simulink model "mdl4"  (Simulink 8.3)
settings: Solver=FixedStepDiscrete  SolverMode=SingleTasking  StartTime=TIME(1)  StopTime=TIME(end)  FixedStep=SIMSTEP  RelTol=1e-3
values from neighbouring files (symbols this model uses):
  Parameter113 = 123    [scr_simdata_all.mat]
  Parameter131 = 3    [scr_simdata_all.mat]
  Parameter132 = 100    [scr_simdata_all.mat]
  Parameter144 = 3    [scr_simdata_all.mat]
  Parameter51 = 0    [scr_simdata_all.mat]
  Parameter52 = 1    [scr_simdata_all.mat]
  Parameter53 = 2    [scr_simdata_all.mat]
  Parameter54 = 255    [scr_simdata_all.mat]
  Parameter69 = 27    [scr_simdata_all.mat]
  Parameter91 = 75    [scr_simdata_all.mat]
  SIMSTEP = 0.0001024    [scr_simdata_all.mat]
(part 3 of 4)

== system mdl4/SubSystem2493/SubSystem2494/SubSystem2500/SubSystem2504/SubSystem2519/SubSystem2528 ==
  note: ***編集禁止***
  element : Inport
  Inside_DSR : DataStoreRead  DataStoreName=DSM127
  Selector : Selector  IndexOptions=Index vector (port)  Indices=[1 3]
  Output : Outport
  wires:
  Inside_DSR/1 -> Selector/1  "mdl4_SubSystem2493_SubSystem2494_SubSystem2500_SubSystem2504_SubSystem2519_SubSystem2528_Inside_DSR_1"
  element/1 -> Selector/2
  Selector/1 -> Output/1  "mdl4_SubSystem2493_SubSystem2494_SubSystem2500_SubSystem2504_SubSystem2519_SubSystem2528_Selector_1"

== system mdl4/SubSystem2493/SubSystem2494/SubSystem2500/SubSystem2504/SubSystem2519/SubSystem2529 ==
  note: ***編集禁止***
  element : Inport
  Inside_DSR : DataStoreRead  DataStoreName=DSM107
  Selector : Selector  IndexOptions=Index vector (port)  Indices=[1 3]
  Output : Outport
  wires:
  Inside_DSR/1 -> Selector/1  "mdl4_SubSystem2493_SubSystem2494_SubSystem2500_SubSystem2504_SubSystem2519_SubSystem2529_Inside_DSR_1"
  element/1 -> Selector/2
  Selector/1 -> Output/1  "mdl4_SubSystem2493_SubSystem2494_SubSystem2500_SubSystem2504_SubSystem2519_SubSystem2529_Selector_1"

== system mdl4/SubSystem2493/SubSystem2494/SubSystem2500/SubSystem2504/SubSystem2519/SubSystem2530 ==
  note: ***編集禁止***
  element : Inport
  Inside_DSR : DataStoreRead  DataStoreName=DSM109
  Selector : Selector  IndexOptions=Index vector (port)  Indices=[1 3]
  Output : Outport
  wires:
  Inside_DSR/1 -> Selector/1  "mdl4_SubSystem2493_SubSystem2494_SubSystem2500_SubSystem2504_SubSystem2519_SubSystem2530_Inside_DSR_1"
  element/1 -> Selector/2
  Selector/1 -> Output/1  "mdl4_SubSystem2493_SubSystem2494_SubSystem2500_SubSystem2504_SubSystem2519_SubSystem2530_Selector_1"

== system mdl4/SubSystem2493/SubSystem2494/SubSystem2500/SubSystem2504/SubSystem2519/SubSystem2531 ==
  note: ***編集禁止***
  element : Inport
  Inside_DSR : DataStoreRead  DataStoreName=DSM103
  Selector : Selector  IndexOptions=Index vector (port)  Indices=[1 3]
  Output : Outport
  wires:
  Inside_DSR/1 -> Selector/1  "mdl4_SubSystem2493_SubSystem2494_SubSystem2500_SubSystem2504_SubSystem2519_SubSystem2531_Inside_DSR_1"
  element/1 -> Selector/2
  Selector/1 -> Output/1  "mdl4_SubSystem2493_SubSystem2494_SubSystem2500_SubSystem2504_SubSystem2519_SubSystem2531_Selector_1"

== system mdl4/SubSystem2493/SubSystem2494/SubSystem2500/SubSystem2504/SubSystem2519/SubSystem2532 ==
  note: ***編集禁止***
  In1 : Inport
  In2 : Inport  Port=2
  RO1 : RelationalOperator  Operator=>  InputSameDT=on
  single1 : DataTypeConversion  OutDataTypeStr=single  SaturateOnIntegerOverflow=on  RndMeth=Zero
  single2 : DataTypeConversion  OutDataTypeStr=single  SaturateOnIntegerOverflow=on  RndMeth=Zero
  Out1 : Outport
  wires:
  single2/1 -> RO1/2  "mdl4_SubSystem2493_SubSystem2494_SubSystem2500_SubSystem2504_SubSystem2519_SubSystem2532_single2_1"
  single1/1 -> RO1/1  "mdl4_SubSystem2493_SubSystem2494_SubSystem2500_SubSystem2504_SubSystem2519_SubSystem2532_single1_1"
  In1/1 -> single1/1
  In2/1 -> single2/1
  RO1/1 -> Out1/1  "mdl4_SubSystem2493_SubSystem2494_SubSystem2500_SubSystem2504_SubSystem2519_SubSystem2532_RO1_1"

== system mdl4/SubSystem2493/SubSystem2494/SubSystem2500/SubSystem2504/SubSystem2533/SubSystem2534 ==
  note: ***編集禁止***
  In1 : Inport
  In2 : Inport  Port=2
  RO1 : RelationalOperator  Operator===  InputSameDT=on
  single1 : DataTypeConversion  OutDataTypeStr=single  SaturateOnIntegerOverflow=on  RndMeth=Zero
  single2 : DataTypeConversion  OutDataTypeStr=single  SaturateOnIntegerOverflow=on  RndMeth=Zero
  Out1 : Outport
  wires:
  RO1/1 -> Out1/1  "mdl4_SubSystem2493_SubSystem2494_SubSystem2500_SubSystem2504_SubSystem2533_SubSystem2534_RO1_1"
  In2/1 -> single2/1
  In1/1 -> single1/1
  single1/1 -> RO1/1  "mdl4_SubSystem2493_SubSystem2494_SubSystem2500_SubSystem2504_SubSystem2533_SubSystem2534_single1_1"
  single2/1 -> RO1/2  "mdl4_SubSystem2493_SubSystem2494_SubSystem2500_SubSystem2504_SubSystem2533_SubSystem2534_single2_1"

== system mdl4/SubSystem2493/SubSystem2494/SubSystem2500/SubSystem2504/SubSystem2533/SubSystem2535 ==
  note: ***編集禁止***
  In1 : Inport
  In2 : Inport  Port=2
  RO1 : RelationalOperator  Operator===  InputSameDT=on
  single1 : DataTypeConversion  OutDataTypeStr=single  SaturateOnIntegerOverflow=on  RndMeth=Zero
  single2 : DataTypeConversion  OutDataTypeStr=single  SaturateOnIntegerOverflow=on  RndMeth=Zero
  Out1 : Outport
  wires:
  RO1/1 -> Out1/1  "mdl4_SubSystem2493_SubSystem2494_SubSystem2500_SubSystem2504_SubSystem2533_SubSystem2535_RO1_1"
  In2/1 -> single2/1
  In1/1 -> single1/1
  single1/1 -> RO1/1  "mdl4_SubSystem2493_SubSystem2494_SubSystem2500_SubSystem2504_SubSystem2533_SubSystem2535_single1_1"
  single2/1 -> RO1/2  "mdl4_SubSystem2493_SubSystem2494_SubSystem2500_SubSystem2504_SubSystem2533_SubSystem2535_single2_1"

== system mdl4/SubSystem2493/SubSystem2494/SubSystem2500/SubSystem2504/SubSystem2533/SubSystem2536 ==
  note: ***編集禁止***
  In1 : Inport
  In2 : Inport  Port=2
  RO1 : RelationalOperator  Operator===  InputSameDT=on
  single1 : DataTypeConversion  OutDataTypeStr=single  SaturateOnIntegerOverflow=on  RndMeth=Zero
  single2 : DataTypeConversion  OutDataTypeStr=single  SaturateOnIntegerOverflow=on  RndMeth=Zero
  Out1 : Outport
  wires:
  RO1/1 -> Out1/1  "mdl4_SubSystem2493_SubSystem2494_SubSystem2500_SubSystem2504_SubSystem2533_SubSystem2536_RO1_1"
  In2/1 -> single2/1
  In1/1 -> single1/1
  single1/1 -> RO1/1  "mdl4_SubSystem2493_SubSystem2494_SubSystem2500_SubSystem2504_SubSystem2533_SubSystem2536_single1_1"
  single2/1 -> RO1/2  "mdl4_SubSystem2493_SubSystem2494_SubSystem2500_SubSystem2504_SubSystem2533_SubSystem2536_single2_1"

== system mdl4/SubSystem2493/SubSystem2494/SubSystem2500/SubSystem2504/SubSystem2533/SubSystem2537 ==
  note: Text638
  note: Text637
  note: Text636
  note: Text635
  Block7601 : Inport
  Block7602 : Inport  Port=2
  Block7603 : EnablePort
  Block7604 : Constant  OutDataTypeStr=double  SampleTime=-1
  Block7605 : Constant  Value=0  OutDataTypeStr=double  SampleTime=-1
  Block7606 : Constant  OutDataTypeStr=double  SampleTime=-1
  Block7607 : DataStoreRead  DataStoreName=DSM294
  Block7608 : DataStoreWrite  DataStoreName=DSM277
  Block7609 : Demux  Outputs=2
  Block7610 : Sum  Inputs=|++  OutDataTypeStr=double  RndMeth=Zero  SaturateOnIntegerOverflow=on  InputSameDT=on
  Block7611 : Sum  Inputs=++|  OutDataTypeStr=double  RndMeth=Zero  SaturateOnIntegerOverflow=on  InputSameDT=on
  Block7612 : Switch  Threshold=0.5  RndMeth=Zero  SaturateOnIntegerOverflow=on  InputSameDT=on
  SubSystem2538 : Subsystem  Priority=10  TreatAsAtomicUnit=on  mask(***ATC.DSWVEC***){bd_version=1.01.A, r0=DSM293, r1=-1, r2=, r3=, r4=, r5=, r6=, r7=, r8=, r9=, c0=, c1=, c2=, c3=, c4=, c5=, c6=, c7=, c8=, c9=}
      mask prompts: bd_version "Version"
      mask help: これはAutoCからのブロックです．編集禁止．
      settings: AttributesFormatString=Attribute1937  OpenFcn=warndlg('変更禁止!');
      mask Help: web(ui_blockhelpmng(gcb));
      mask Display: disp('ATC.DSRVEC')
  SubSystem2539 : Subsystem  Priority=10  TreatAsAtomicUnit=on  mask(***ATC.DSWVEC***){bd_version=1.01.A, r0=DSM295, r1=-1, r2=, r3=, r4=, r5=, r6=, r7=, r8=, r9=, c0=, c1=, c2=, c3=, c4=, c5=, c6=, c7=, c8=, c9=}
      mask prompts: bd_version "Version"
      mask help: これはAutoCからのブロックです．編集禁止．
      settings: AttributesFormatString=Attribute1938  OpenFcn=warndlg('変更禁止!');
      mask Help: web(ui_blockhelpmng(gcb));
      mask Display: disp('ATC.DSRVEC')
  SubSystem2540 : Subsystem
  wires:
  Block7602/1 -> Block7610/1, Block7611/2
  Block7601/1 -> Block7609/1
  Block7609/1 -> SubSystem2538/1(input)
  Block7609/2 -> SubSystem2539/1(input)
  Block7604/1 -> Block7610/2  "mdl4_SubSystem2493_SubSystem2494_SubSystem2500_SubSystem2504_SubSystem2533_SubSystem2537_Block7604_1"
  Block7610/1 -> SubSystem2538/2(element), SubSystem2539/2(element)  "mdl4_SubSystem2493_SubSystem2494_SubSystem2500_SubSystem2504_SubSystem2533_SubSystem2537_Block7610_1"
  Block7607/1 -> SubSystem2540/2(In2)  "mdl4_SubSystem2493_SubSystem2494_SubSystem2500_SubSystem2504_SubSystem2533_SubSystem2537_Block7607_1"
  Block7606/1 -> Block7611/1  "mdl4_SubSystem2493_SubSystem2494_SubSystem2500_SubSystem2504_SubSystem2533_SubSystem2537_Block7606_1"
  SubSystem2540/1(Out1) -> Block7612/2
  Block7612/1 -> Block7608/1  "mdl4_SubSystem2493_SubSystem2494_SubSystem2500_SubSystem2504_SubSystem2533_SubSystem2537_Block7612_1"
  Block7611/1 -> Block7612/3, SubSystem2540/1(In1)  "mdl4_SubSystem2493_SubSystem2494_SubSystem2500_SubSystem2504_SubSystem2533_SubSystem2537_Block7611_1"
  Block7605/1 -> Block7612/1  "mdl4_SubSystem2493_SubSystem2494_SubSystem2500_SubSystem2504_SubSystem2533_SubSystem2537_Block7605_1"

== system mdl4/SubSystem2493/SubSystem2494/SubSystem2500/SubSystem2504/SubSystem2533/SubSystem2541 ==
  note: Text639
  Block7613 : Inport
  Block7614 : Inport  Port=2
  Block7615 : EnablePort
  Block7616 : Constant  OutDataTypeStr=double  SampleTime=-1
  Block7617 : Demux  Outputs=2
  Block7618 : Sum  Inputs=|++  OutDataTypeStr=double  RndMeth=Zero  SaturateOnIntegerOverflow=on  InputSameDT=on
  SubSystem2542 : Subsystem  Priority=10  TreatAsAtomicUnit=on  mask(***ATC.DSWVEC***){bd_version=1.01.A, r0=DSM279, r1=-1, r2=, r3=, r4=, r5=, r6=, r7=, r8=, r9=, c0=, c1=, c2=, c3=, c4=, c5=, c6=, c7=, c8=, c9=}
      mask prompts: bd_version "Version"
      mask help: これはAutoCからのブロックです．編集禁止．
      settings: AttributesFormatString=Attribute1941  OpenFcn=warndlg('変更禁止!');
      mask Help: web(ui_blockhelpmng(gcb));
      mask Display: disp('ATC.DSRVEC')
  SubSystem2543 : Subsystem  Priority=10  TreatAsAtomicUnit=on  mask(***ATC.DSWVEC***){bd_version=1.01.A, r0=DSM280, r1=-1, r2=, r3=, r4=, r5=, r6=, r7=, r8=, r9=, c0=, c1=, c2=, c3=, c4=, c5=, c6=, c7=, c8=, c9=}
      mask prompts: bd_version "Version"
      mask help: これはAutoCからのブロックです．編集禁止．
      settings: AttributesFormatString=Attribute1942  OpenFcn=warndlg('変更禁止!');
      mask Help: web(ui_blockhelpmng(gcb));
      mask Display: disp('ATC.DSRVEC')
  wires:
  Block7613/1 -> Block7617/1
  Block7617/1 -> SubSystem2542/1(input)
  Block7617/2 -> SubSystem2543/1(input)
  Block7616/1 -> Block7618/2  "mdl4_SubSystem2493_SubSystem2494_SubSystem2500_SubSystem2504_SubSystem2533_SubSystem2541_Block7616_1"
  Block7614/1 -> Block7618/1
  Block7618/1 -> SubSystem2542/2(element), SubSystem2543/2(element)  "mdl4_SubSystem2493_SubSystem2494_SubSystem2500_SubSystem2504_SubSystem2533_SubSystem2541_Block7618_1"

== system mdl4/SubSystem2493/SubSystem2494/SubSystem2500/SubSystem2504/SubSystem2533/SubSystem2544 ==
  note: Text640
  Block7619 : Inport
  Block7620 : Inport  Port=2
  Block7621 : EnablePort
  Block7622 : Constant  OutDataTypeStr=double  SampleTime=-1
  Block7623 : Demux  Outputs=2
  Block7624 : Sum  Inputs=|++  OutDataTypeStr=double  RndMeth=Zero  SaturateOnIntegerOverflow=on  InputSameDT=on
  SubSystem2545 : Subsystem  Priority=10  TreatAsAtomicUnit=on  mask(***ATC.DSWVEC***){bd_version=1.01.A, r0=DSM281, r1=-1, r2=, r3=, r4=, r5=, r6=, r7=, r8=, r9=, c0=, c1=, c2=, c3=, c4=, c5=, c6=, c7=, c8=, c9=}
      mask prompts: bd_version "Version"
      mask help: これはAutoCからのブロックです．編集禁止．
      settings: AttributesFormatString=Attribute1945  OpenFcn=warndlg('変更禁止!');
      mask Help: web(ui_blockhelpmng(gcb));
      mask Display: disp('ATC.DSRVEC')
  SubSystem2546 : Subsystem  Priority=10  TreatAsAtomicUnit=on  mask(***ATC.DSWVEC***){bd_version=1.01.A, r0=DSM282, r1=-1, r2=, r3=, r4=, r5=, r6=, r7=, r8=, r9=, c0=, c1=, c2=, c3=, c4=, c5=, c6=, c7=, c8=, c9=}
      mask prompts: bd_version "Version"
      mask help: これはAutoCからのブロックです．編集禁止．
      settings: AttributesFormatString=Attribute1946  OpenFcn=warndlg('変更禁止!');
      mask Help: web(ui_blockhelpmng(gcb));
      mask Display: disp('ATC.DSRVEC')
  wires:
  Block7619/1 -> Block7623/1
  Block7623/1 -> SubSystem2545/1(input)
  Block7623/2 -> SubSystem2546/1(input)
  Block7622/1 -> Block7624/2  "mdl4_SubSystem2493_SubSystem2494_SubSystem2500_SubSystem2504_SubSystem2533_SubSystem2544_Block7622_1"
  Block7620/1 -> Block7624/1
  Block7624/1 -> SubSystem2545/2(element), SubSystem2546/2(element)  "mdl4_SubSystem2493_SubSystem2494_SubSystem2500_SubSystem2504_SubSystem2533_SubSystem2544_Block7624_1"

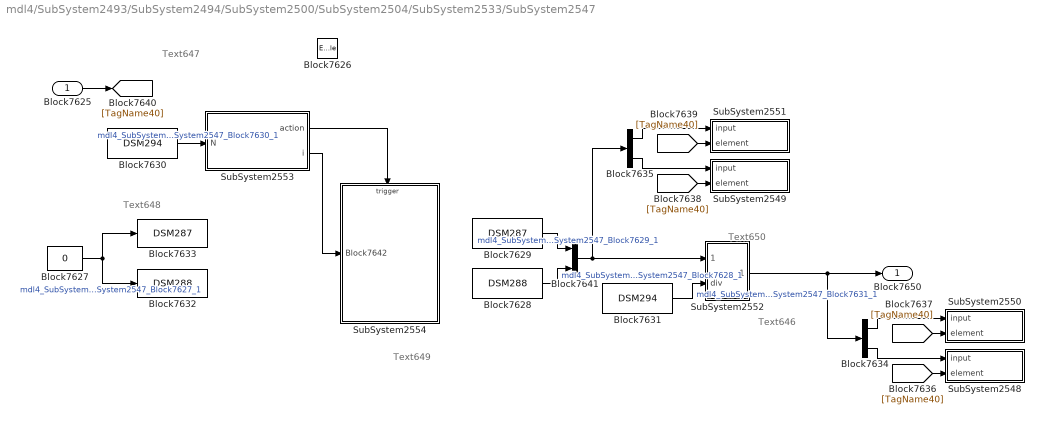
== system mdl4/SubSystem2493/SubSystem2494/SubSystem2500/SubSystem2504/SubSystem2533/SubSystem2547 ==
  note: Text650
  note: Text649
  note: Text648
  note: Text647
  note: Text646
  Block7625 : Inport
  Block7626 : EnablePort
  Block7627 : Constant  Value=0  OutDataTypeStr=double  SampleTime=-1
  Block7628 : DataStoreRead  Priority=30  DataStoreName=DSM288
      settings: AttributesFormatString=Attribute1949
  Block7629 : DataStoreRead  Priority=30  DataStoreName=DSM287
      settings: AttributesFormatString=Attribute1950
  Block7630 : DataStoreRead  DataStoreName=DSM294
  Block7631 : DataStoreRead  DataStoreName=DSM294
  Block7632 : DataStoreWrite  Priority=10  DataStoreName=DSM288
      settings: AttributesFormatString=Attribute1951
  Block7633 : DataStoreWrite  Priority=10  DataStoreName=DSM287
      settings: AttributesFormatString=Attribute1952
  Block7634 : Demux  Outputs=2
  Block7635 : Demux  Outputs=2
  Block7641 : Mux  Inputs=2
  SubSystem2548 : Subsystem  TreatAsAtomicUnit=on  mask(***ATC.DSWVEC***){bd_version=1.01.A, r0=DSM290, r1=-1, r2=, r3=, r4=, r5=, r6=, r7=, r8=, r9=, c0=, c1=, c2=, c3=, c4=, c5=, c6=, c7=, c8=, c9=}
      mask prompts: bd_version "Version"
      mask help: これはAutoCからのブロックです．編集禁止．
      settings: OpenFcn=warndlg('変更禁止!');
      mask Help: web(ui_blockhelpmng(gcb));
      mask Display: disp('ATC.DSRVEC')
  SubSystem2549 : Subsystem  TreatAsAtomicUnit=on  mask(***ATC.DSWVEC***){bd_version=1.01.A, r0=DSM292, r1=-1, r2=, r3=, r4=, r5=, r6=, r7=, r8=, r9=, c0=, c1=, c2=, c3=, c4=, c5=, c6=, c7=, c8=, c9=}
      mask prompts: bd_version "Version"
      mask help: これはAutoCからのブロックです．編集禁止．
      settings: OpenFcn=warndlg('変更禁止!');
      mask Help: web(ui_blockhelpmng(gcb));
      mask Display: disp('ATC.DSRVEC')
  SubSystem2550 : Subsystem  TreatAsAtomicUnit=on  mask(***ATC.DSWVEC***){bd_version=1.01.A, r0=DSM289, r1=-1, r2=, r3=, r4=, r5=, r6=, r7=, r8=, r9=, c0=, c1=, c2=, c3=, c4=, c5=, c6=, c7=, c8=, c9=}
      mask prompts: bd_version "Version"
      mask help: これはAutoCからのブロックです．編集禁止．
      settings: OpenFcn=warndlg('変更禁止!');
      mask Help: web(ui_blockhelpmng(gcb));
      mask Display: disp('ATC.DSRVEC')
  SubSystem2551 : Subsystem  TreatAsAtomicUnit=on  mask(***ATC.DSWVEC***){bd_version=1.01.A, r0=DSM291, r1=-1, r2=, r3=, r4=, r5=, r6=, r7=, r8=, r9=, c0=, c1=, c2=, c3=, c4=, c5=, c6=, c7=, c8=, c9=}
      mask prompts: bd_version "Version"
      mask help: これはAutoCからのブロックです．編集禁止．
      settings: OpenFcn=warndlg('変更禁止!');
      mask Help: web(ui_blockhelpmng(gcb));
      mask Display: disp('ATC.DSRVEC')
  SubSystem2552 : Subsystem  TreatAsAtomicUnit=on  mask(***ATC.DIVISION***){bd_version=1.01.A, r0=チェック無し, r1=, r2=, r3=, r4=, r5=, r6=, r7=, r8=, r9=, c0=, c1=, c2=, c3=, c4=, c5=, c6=, c7=, c8=, c9=}
      mask prompts: bd_version "Version"
      mask help: これはAutoCからのブロックです．編集禁止．
      settings: OpenFcn=warndlg('変更禁止!');
      mask Help: web(ui_blockhelpmng(gcb));
  SubSystem2553 : Subsystem  Priority=20  TreatAsAtomicUnit=on  mask(***ATC.ITERATOR***){}
      mask help: これはAutoCからのブロックです．編集禁止．
      settings: AttributesFormatString=Attribute1953  OpenFcn=warndlg('変更禁止!');  RTWSystemCode=Inline
  SubSystem2554 : Subsystem  TreatAsAtomicUnit=on
  Block7650 : Outport
  wires:
  Block7627/1 -> Block7632/1, Block7633/1  "mdl4_SubSystem2493_SubSystem2494_SubSystem2500_SubSystem2504_SubSystem2533_SubSystem2547_Block7627_1"
  Block7635/2 -> SubSystem2549/1(input)
  [TagName40] -> SubSystem2549/2(element)
  Block7635/1 -> SubSystem2551/1(input)
  [TagName40] -> SubSystem2551/2(element)
  Block7634/2 -> SubSystem2548/1(input)
  [TagName40] -> SubSystem2548/2(element)
  Block7634/1 -> SubSystem2550/1(input)
  [TagName40] -> SubSystem2550/2(element)
  Block7641/1 -> Block7635/1, SubSystem2552/1(mult)
  Block7628/1 -> Block7641/2  "mdl4_SubSystem2493_SubSystem2494_SubSystem2500_SubSystem2504_SubSystem2533_SubSystem2547_Block7628_1"
  Block7629/1 -> Block7641/1  "mdl4_SubSystem2493_SubSystem2494_SubSystem2500_SubSystem2504_SubSystem2533_SubSystem2547_Block7629_1"
  SubSystem2552/1(Out) -> Block7634/1, Block7650/1
  Block7631/1 -> SubSystem2552/2(div)  "mdl4_SubSystem2493_SubSystem2494_SubSystem2500_SubSystem2504_SubSystem2533_SubSystem2547_Block7631_1"
  SubSystem2553/2(i) -> SubSystem2554/1(Block7642)
  SubSystem2553/1(action) -> SubSystem2554/Trigger
  Block7630/1 -> SubSystem2553/1(N)  "mdl4_SubSystem2493_SubSystem2494_SubSystem2500_SubSystem2504_SubSystem2533_SubSystem2547_Block7630_1"
  Block7625/1 -> [TagName40]

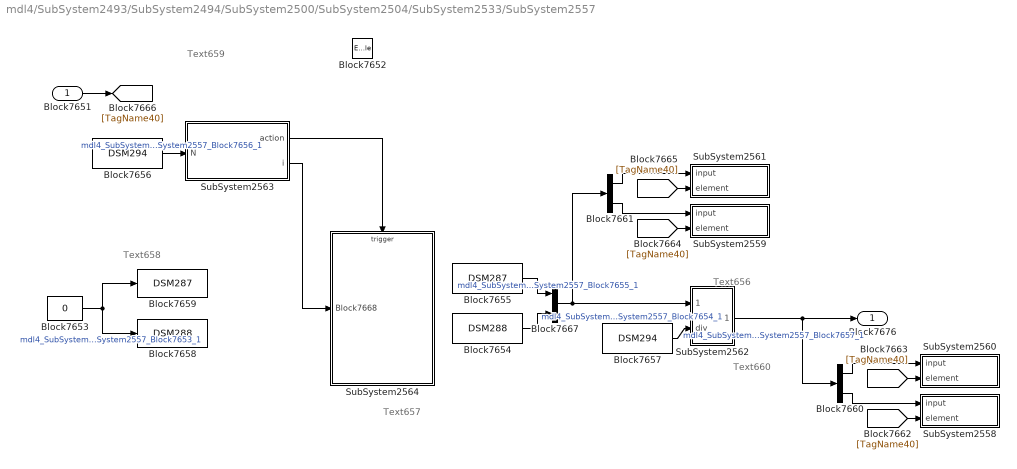
== system mdl4/SubSystem2493/SubSystem2494/SubSystem2500/SubSystem2504/SubSystem2533/SubSystem2557 ==
  note: Text660
  note: Text659
  note: Text658
  note: Text657
  note: Text656
  Block7651 : Inport
  Block7652 : EnablePort
  Block7653 : Constant  Value=0  OutDataTypeStr=double  SampleTime=-1
  Block7654 : DataStoreRead  Priority=30  DataStoreName=DSM288
      settings: AttributesFormatString=Attribute1956
  Block7655 : DataStoreRead  Priority=30  DataStoreName=DSM287
      settings: AttributesFormatString=Attribute1957
  Block7656 : DataStoreRead  DataStoreName=DSM294
  Block7657 : DataStoreRead  DataStoreName=DSM294
  Block7658 : DataStoreWrite  Priority=10  DataStoreName=DSM288
      settings: AttributesFormatString=Attribute1958
  Block7659 : DataStoreWrite  Priority=10  DataStoreName=DSM287
      settings: AttributesFormatString=Attribute1959
  Block7660 : Demux  Outputs=2
  Block7661 : Demux  Outputs=2
  Block7667 : Mux  Inputs=2
  SubSystem2558 : Subsystem  TreatAsAtomicUnit=on  mask(***ATC.DSWVEC***){bd_version=1.01.A, r0=DSM290, r1=-1, r2=, r3=, r4=, r5=, r6=, r7=, r8=, r9=, c0=, c1=, c2=, c3=, c4=, c5=, c6=, c7=, c8=, c9=}
      mask prompts: bd_version "Version"
      mask help: これはAutoCからのブロックです．編集禁止．
      settings: OpenFcn=warndlg('変更禁止!');
      mask Help: web(ui_blockhelpmng(gcb));
      mask Display: disp('ATC.DSRVEC')
  SubSystem2559 : Subsystem  TreatAsAtomicUnit=on  mask(***ATC.DSWVEC***){bd_version=1.01.A, r0=DSM292, r1=-1, r2=, r3=, r4=, r5=, r6=, r7=, r8=, r9=, c0=, c1=, c2=, c3=, c4=, c5=, c6=, c7=, c8=, c9=}
      mask prompts: bd_version "Version"
      mask help: これはAutoCからのブロックです．編集禁止．
      settings: OpenFcn=warndlg('変更禁止!');
      mask Help: web(ui_blockhelpmng(gcb));
      mask Display: disp('ATC.DSRVEC')
  SubSystem2560 : Subsystem  TreatAsAtomicUnit=on  mask(***ATC.DSWVEC***){bd_version=1.01.A, r0=DSM289, r1=-1, r2=, r3=, r4=, r5=, r6=, r7=, r8=, r9=, c0=, c1=, c2=, c3=, c4=, c5=, c6=, c7=, c8=, c9=}
      mask prompts: bd_version "Version"
      mask help: これはAutoCからのブロックです．編集禁止．
      settings: OpenFcn=warndlg('変更禁止!');
      mask Help: web(ui_blockhelpmng(gcb));
      mask Display: disp('ATC.DSRVEC')
  SubSystem2561 : Subsystem  TreatAsAtomicUnit=on  mask(***ATC.DSWVEC***){bd_version=1.01.A, r0=DSM291, r1=-1, r2=, r3=, r4=, r5=, r6=, r7=, r8=, r9=, c0=, c1=, c2=, c3=, c4=, c5=, c6=, c7=, c8=, c9=}
      mask prompts: bd_version "Version"
      mask help: これはAutoCからのブロックです．編集禁止．
      settings: OpenFcn=warndlg('変更禁止!');
      mask Help: web(ui_blockhelpmng(gcb));
      mask Display: disp('ATC.DSRVEC')
  SubSystem2562 : Subsystem  TreatAsAtomicUnit=on  mask(***ATC.DIVISION***){bd_version=1.01.A, r0=チェック無し, r1=, r2=, r3=, r4=, r5=, r6=, r7=, r8=, r9=, c0=, c1=, c2=, c3=, c4=, c5=, c6=, c7=, c8=, c9=}
      mask prompts: bd_version "Version"
      mask help: これはAutoCからのブロックです．編集禁止．
      settings: OpenFcn=warndlg('変更禁止!');
      mask Help: web(ui_blockhelpmng(gcb));
  SubSystem2563 : Subsystem  Priority=20  TreatAsAtomicUnit=on  mask(***ATC.ITERATOR***){}
      mask help: これはAutoCからのブロックです．編集禁止．
      settings: AttributesFormatString=Attribute1960  OpenFcn=warndlg('変更禁止!');  RTWSystemCode=Inline
  SubSystem2564 : Subsystem  TreatAsAtomicUnit=on
  Block7676 : Outport
  wires:
  Block7656/1 -> SubSystem2563/1(N)  "mdl4_SubSystem2493_SubSystem2494_SubSystem2500_SubSystem2504_SubSystem2533_SubSystem2557_Block7656_1"
  SubSystem2563/1(action) -> SubSystem2564/Trigger
  SubSystem2563/2(i) -> SubSystem2564/1(Block7668)
  Block7657/1 -> SubSystem2562/2(div)  "mdl4_SubSystem2493_SubSystem2494_SubSystem2500_SubSystem2504_SubSystem2533_SubSystem2557_Block7657_1"
  SubSystem2562/1(Out) -> Block7676/1, Block7660/1
  Block7655/1 -> Block7667/1  "mdl4_SubSystem2493_SubSystem2494_SubSystem2500_SubSystem2504_SubSystem2533_SubSystem2557_Block7655_1"
  Block7654/1 -> Block7667/2  "mdl4_SubSystem2493_SubSystem2494_SubSystem2500_SubSystem2504_SubSystem2533_SubSystem2557_Block7654_1"
  Block7667/1 -> Block7661/1, SubSystem2562/1(mult)
  [TagName40] -> SubSystem2560/2(element)
  Block7660/1 -> SubSystem2560/1(input)
  [TagName40] -> SubSystem2558/2(element)
  Block7660/2 -> SubSystem2558/1(input)
  [TagName40] -> SubSystem2561/2(element)
  Block7661/1 -> SubSystem2561/1(input)
  [TagName40] -> SubSystem2559/2(element)
  Block7661/2 -> SubSystem2559/1(input)
  Block7653/1 -> Block7659/1, Block7658/1  "mdl4_SubSystem2493_SubSystem2494_SubSystem2500_SubSystem2504_SubSystem2533_SubSystem2557_Block7653_1"
  Block7651/1 -> [TagName40]

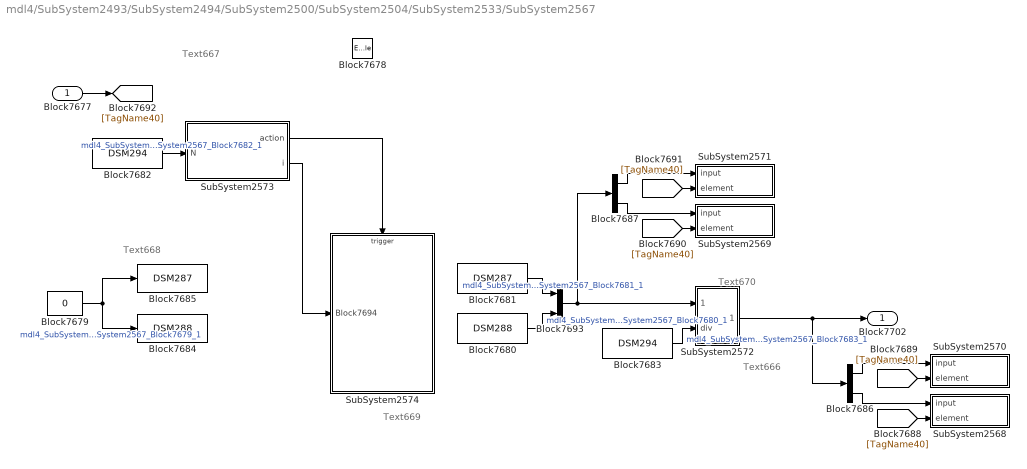
== system mdl4/SubSystem2493/SubSystem2494/SubSystem2500/SubSystem2504/SubSystem2533/SubSystem2567 ==
  note: Text670
  note: Text669
  note: Text668
  note: Text667
  note: Text666
  Block7677 : Inport
  Block7678 : EnablePort
  Block7679 : Constant  Value=0  OutDataTypeStr=double  SampleTime=-1
  Block7680 : DataStoreRead  Priority=30  DataStoreName=DSM288
      settings: AttributesFormatString=Attribute1963
  Block7681 : DataStoreRead  Priority=30  DataStoreName=DSM287
      settings: AttributesFormatString=Attribute1964
  Block7682 : DataStoreRead  DataStoreName=DSM294
  Block7683 : DataStoreRead  DataStoreName=DSM294
  Block7684 : DataStoreWrite  Priority=10  DataStoreName=DSM288
      settings: AttributesFormatString=Attribute1965
  Block7685 : DataStoreWrite  Priority=10  DataStoreName=DSM287
      settings: AttributesFormatString=Attribute1966
  Block7686 : Demux  Outputs=2
  Block7687 : Demux  Outputs=2
  Block7693 : Mux  Inputs=2
  SubSystem2568 : Subsystem  TreatAsAtomicUnit=on  mask(***ATC.DSWVEC***){bd_version=1.01.A, r0=DSM290, r1=-1, r2=, r3=, r4=, r5=, r6=, r7=, r8=, r9=, c0=, c1=, c2=, c3=, c4=, c5=, c6=, c7=, c8=, c9=}
      mask prompts: bd_version "Version"
      mask help: これはAutoCからのブロックです．編集禁止．
      settings: OpenFcn=warndlg('変更禁止!');
      mask Help: web(ui_blockhelpmng(gcb));
      mask Display: disp('ATC.DSRVEC')
  SubSystem2569 : Subsystem  TreatAsAtomicUnit=on  mask(***ATC.DSWVEC***){bd_version=1.01.A, r0=DSM292, r1=-1, r2=, r3=, r4=, r5=, r6=, r7=, r8=, r9=, c0=, c1=, c2=, c3=, c4=, c5=, c6=, c7=, c8=, c9=}
      mask prompts: bd_version "Version"
      mask help: これはAutoCからのブロックです．編集禁止．
      settings: OpenFcn=warndlg('変更禁止!');
      mask Help: web(ui_blockhelpmng(gcb));
      mask Display: disp('ATC.DSRVEC')
  SubSystem2570 : Subsystem  TreatAsAtomicUnit=on  mask(***ATC.DSWVEC***){bd_version=1.01.A, r0=DSM289, r1=-1, r2=, r3=, r4=, r5=, r6=, r7=, r8=, r9=, c0=, c1=, c2=, c3=, c4=, c5=, c6=, c7=, c8=, c9=}
      mask prompts: bd_version "Version"
      mask help: これはAutoCからのブロックです．編集禁止．
      settings: OpenFcn=warndlg('変更禁止!');
      mask Help: web(ui_blockhelpmng(gcb));
      mask Display: disp('ATC.DSRVEC')
  SubSystem2571 : Subsystem  TreatAsAtomicUnit=on  mask(***ATC.DSWVEC***){bd_version=1.01.A, r0=DSM291, r1=-1, r2=, r3=, r4=, r5=, r6=, r7=, r8=, r9=, c0=, c1=, c2=, c3=, c4=, c5=, c6=, c7=, c8=, c9=}
      mask prompts: bd_version "Version"
      mask help: これはAutoCからのブロックです．編集禁止．
      settings: OpenFcn=warndlg('変更禁止!');
      mask Help: web(ui_blockhelpmng(gcb));
      mask Display: disp('ATC.DSRVEC')
  SubSystem2572 : Subsystem  TreatAsAtomicUnit=on  mask(***ATC.DIVISION***){bd_version=1.01.A, r0=チェック無し, r1=, r2=, r3=, r4=, r5=, r6=, r7=, r8=, r9=, c0=, c1=, c2=, c3=, c4=, c5=, c6=, c7=, c8=, c9=}
      mask prompts: bd_version "Version"
      mask help: これはAutoCからのブロックです．編集禁止．
      settings: OpenFcn=warndlg('変更禁止!');
      mask Help: web(ui_blockhelpmng(gcb));
  SubSystem2573 : Subsystem  Priority=20  TreatAsAtomicUnit=on  mask(***ATC.ITERATOR***){}
      mask help: これはAutoCからのブロックです．編集禁止．
      settings: AttributesFormatString=Attribute1967  OpenFcn=warndlg('変更禁止!');  RTWSystemCode=Inline
  SubSystem2574 : Subsystem  TreatAsAtomicUnit=on
  Block7702 : Outport
  wires:
  Block7679/1 -> Block7684/1, Block7685/1  "mdl4_SubSystem2493_SubSystem2494_SubSystem2500_SubSystem2504_SubSystem2533_SubSystem2567_Block7679_1"
  Block7687/2 -> SubSystem2569/1(input)
  [TagName40] -> SubSystem2569/2(element)
  Block7687/1 -> SubSystem2571/1(input)
  [TagName40] -> SubSystem2571/2(element)
  Block7686/2 -> SubSystem2568/1(input)
  [TagName40] -> SubSystem2568/2(element)
  Block7686/1 -> SubSystem2570/1(input)
  [TagName40] -> SubSystem2570/2(element)
  Block7693/1 -> Block7687/1, SubSystem2572/1(mult)
  Block7680/1 -> Block7693/2  "mdl4_SubSystem2493_SubSystem2494_SubSystem2500_SubSystem2504_SubSystem2533_SubSystem2567_Block7680_1"
  Block7681/1 -> Block7693/1  "mdl4_SubSystem2493_SubSystem2494_SubSystem2500_SubSystem2504_SubSystem2533_SubSystem2567_Block7681_1"
  SubSystem2572/1(Out) -> Block7686/1, Block7702/1
  Block7683/1 -> SubSystem2572/2(div)  "mdl4_SubSystem2493_SubSystem2494_SubSystem2500_SubSystem2504_SubSystem2533_SubSystem2567_Block7683_1"
  SubSystem2573/2(i) -> SubSystem2574/1(Block7694)
  SubSystem2573/1(action) -> SubSystem2574/Trigger
  Block7682/1 -> SubSystem2573/1(N)  "mdl4_SubSystem2493_SubSystem2494_SubSystem2500_SubSystem2504_SubSystem2533_SubSystem2567_Block7682_1"
  Block7677/1 -> [TagName40]

== system mdl4/SubSystem2493/SubSystem2494/SubSystem2500/SubSystem2504/SubSystem2533/SubSystem2537/SubSystem2538 ==
  note: ***編集禁止***
  input : Inport
  element : Inport  Port=2
  Assignment : Assignment  IndexOptions=Index vector (port)  OutputSizes=[1 1]
  Inside_DSR : DataStoreRead  DataStoreName=DSM293
  Inside_DSW : DataStoreWrite  DataStoreName=DSM293
  wires:
  Assignment/1 -> Inside_DSW/1  "mdl4_SubSystem2493_SubSystem2494_SubSystem2500_SubSystem2504_SubSystem2533_SubSystem2537_SubSystem2538_Assignment_1"
  Inside_DSR/1 -> Assignment/1  "mdl4_SubSystem2493_SubSystem2494_SubSystem2500_SubSystem2504_SubSystem2533_SubSystem2537_SubSystem2538_Inside_DSR_1"
  input/1 -> Assignment/2
  element/1 -> Assignment/3

== system mdl4/SubSystem2493/SubSystem2494/SubSystem2500/SubSystem2504/SubSystem2533/SubSystem2537/SubSystem2539 ==
  note: ***編集禁止***
  input : Inport
  element : Inport  Port=2
  Assignment : Assignment  IndexOptions=Index vector (port)  OutputSizes=[1 1]
  Inside_DSR : DataStoreRead  DataStoreName=DSM295
  Inside_DSW : DataStoreWrite  DataStoreName=DSM295
  wires:
  Assignment/1 -> Inside_DSW/1  "mdl4_SubSystem2493_SubSystem2494_SubSystem2500_SubSystem2504_SubSystem2533_SubSystem2537_SubSystem2539_Assignment_1"
  Inside_DSR/1 -> Assignment/1  "mdl4_SubSystem2493_SubSystem2494_SubSystem2500_SubSystem2504_SubSystem2533_SubSystem2537_SubSystem2539_Inside_DSR_1"
  input/1 -> Assignment/2
  element/1 -> Assignment/3

== system mdl4/SubSystem2493/SubSystem2494/SubSystem2500/SubSystem2504/SubSystem2533/SubSystem2537/SubSystem2540 ==
  note: ***編集禁止***
  In1 : Inport
  In2 : Inport  Port=2
  RO1 : RelationalOperator  Operator===  InputSameDT=on
  single1 : DataTypeConversion  OutDataTypeStr=single  SaturateOnIntegerOverflow=on  RndMeth=Zero
  single2 : DataTypeConversion  OutDataTypeStr=single  SaturateOnIntegerOverflow=on  RndMeth=Zero
  Out1 : Outport
  wires:
  single2/1 -> RO1/2  "mdl4_SubSystem2493_SubSystem2494_SubSystem2500_SubSystem2504_SubSystem2533_SubSystem2537_SubSystem2540_single2_1"
  single1/1 -> RO1/1  "mdl4_SubSystem2493_SubSystem2494_SubSystem2500_SubSystem2504_SubSystem2533_SubSystem2537_SubSystem2540_single1_1"
  In1/1 -> single1/1
  In2/1 -> single2/1
  RO1/1 -> Out1/1  "mdl4_SubSystem2493_SubSystem2494_SubSystem2500_SubSystem2504_SubSystem2533_SubSystem2537_SubSystem2540_RO1_1"

== system mdl4/SubSystem2493/SubSystem2494/SubSystem2500/SubSystem2504/SubSystem2533/SubSystem2541/SubSystem2542 ==
  note: ***編集禁止***
  input : Inport
  element : Inport  Port=2
  Assignment : Assignment  IndexOptions=Index vector (port)  OutputSizes=[1 1]
  Inside_DSR : DataStoreRead  DataStoreName=DSM279
  Inside_DSW : DataStoreWrite  DataStoreName=DSM279
  wires:
  Assignment/1 -> Inside_DSW/1  "mdl4_SubSystem2493_SubSystem2494_SubSystem2500_SubSystem2504_SubSystem2533_SubSystem2541_SubSystem2542_Assignment_1"
  Inside_DSR/1 -> Assignment/1  "mdl4_SubSystem2493_SubSystem2494_SubSystem2500_SubSystem2504_SubSystem2533_SubSystem2541_SubSystem2542_Inside_DSR_1"
  input/1 -> Assignment/2
  element/1 -> Assignment/3

== system mdl4/SubSystem2493/SubSystem2494/SubSystem2500/SubSystem2504/SubSystem2533/SubSystem2541/SubSystem2543 ==
  note: ***編集禁止***
  input : Inport
  element : Inport  Port=2
  Assignment : Assignment  IndexOptions=Index vector (port)  OutputSizes=[1 1]
  Inside_DSR : DataStoreRead  DataStoreName=DSM280
  Inside_DSW : DataStoreWrite  DataStoreName=DSM280
  wires:
  Assignment/1 -> Inside_DSW/1  "mdl4_SubSystem2493_SubSystem2494_SubSystem2500_SubSystem2504_SubSystem2533_SubSystem2541_SubSystem2543_Assignment_1"
  Inside_DSR/1 -> Assignment/1  "mdl4_SubSystem2493_SubSystem2494_SubSystem2500_SubSystem2504_SubSystem2533_SubSystem2541_SubSystem2543_Inside_DSR_1"
  input/1 -> Assignment/2
  element/1 -> Assignment/3

== system mdl4/SubSystem2493/SubSystem2494/SubSystem2500/SubSystem2504/SubSystem2533/SubSystem2544/SubSystem2545 ==
  note: ***編集禁止***
  input : Inport
  element : Inport  Port=2
  Assignment : Assignment  IndexOptions=Index vector (port)  OutputSizes=[1 1]
  Inside_DSR : DataStoreRead  DataStoreName=DSM281
  Inside_DSW : DataStoreWrite  DataStoreName=DSM281
  wires:
  Assignment/1 -> Inside_DSW/1  "mdl4_SubSystem2493_SubSystem2494_SubSystem2500_SubSystem2504_SubSystem2533_SubSystem2544_SubSystem2545_Assignment_1"
  Inside_DSR/1 -> Assignment/1  "mdl4_SubSystem2493_SubSystem2494_SubSystem2500_SubSystem2504_SubSystem2533_SubSystem2544_SubSystem2545_Inside_DSR_1"
  input/1 -> Assignment/2
  element/1 -> Assignment/3

== system mdl4/SubSystem2493/SubSystem2494/SubSystem2500/SubSystem2504/SubSystem2533/SubSystem2544/SubSystem2546 ==
  note: ***編集禁止***
  input : Inport
  element : Inport  Port=2
  Assignment : Assignment  IndexOptions=Index vector (port)  OutputSizes=[1 1]
  Inside_DSR : DataStoreRead  DataStoreName=DSM282
  Inside_DSW : DataStoreWrite  DataStoreName=DSM282
  wires:
  Assignment/1 -> Inside_DSW/1  "mdl4_SubSystem2493_SubSystem2494_SubSystem2500_SubSystem2504_SubSystem2533_SubSystem2544_SubSystem2546_Assignment_1"
  Inside_DSR/1 -> Assignment/1  "mdl4_SubSystem2493_SubSystem2494_SubSystem2500_SubSystem2504_SubSystem2533_SubSystem2544_SubSystem2546_Inside_DSR_1"
  input/1 -> Assignment/2
  element/1 -> Assignment/3

== system mdl4/SubSystem2493/SubSystem2494/SubSystem2500/SubSystem2504/SubSystem2533/SubSystem2547/SubSystem2548 ==
  note: ***編集禁止***
  input : Inport
  element : Inport  Port=2
  Assignment : Assignment  IndexOptions=Index vector (port)  OutputSizes=[1 1]
  Inside_DSR : DataStoreRead  DataStoreName=DSM290
  Inside_DSW : DataStoreWrite  DataStoreName=DSM290
  wires:
  Assignment/1 -> Inside_DSW/1  "mdl4_SubSystem2493_SubSystem2494_SubSystem2500_SubSystem2504_SubSystem2533_SubSystem2547_SubSystem2548_Assignment_1"
  Inside_DSR/1 -> Assignment/1  "mdl4_SubSystem2493_SubSystem2494_SubSystem2500_SubSystem2504_SubSystem2533_SubSystem2547_SubSystem2548_Inside_DSR_1"
  input/1 -> Assignment/2
  element/1 -> Assignment/3

== system mdl4/SubSystem2493/SubSystem2494/SubSystem2500/SubSystem2504/SubSystem2533/SubSystem2547/SubSystem2549 ==
  note: ***編集禁止***
  input : Inport
  element : Inport  Port=2
  Assignment : Assignment  IndexOptions=Index vector (port)  OutputSizes=[1 1]
  Inside_DSR : DataStoreRead  DataStoreName=DSM292
  Inside_DSW : DataStoreWrite  DataStoreName=DSM292
  wires:
  element/1 -> Assignment/3
  input/1 -> Assignment/2
  Inside_DSR/1 -> Assignment/1  "mdl4_SubSystem2493_SubSystem2494_SubSystem2500_SubSystem2504_SubSystem2533_SubSystem2547_SubSystem2549_Inside_DSR_1"
  Assignment/1 -> Inside_DSW/1  "mdl4_SubSystem2493_SubSystem2494_SubSystem2500_SubSystem2504_SubSystem2533_SubSystem2547_SubSystem2549_Assignment_1"

== system mdl4/SubSystem2493/SubSystem2494/SubSystem2500/SubSystem2504/SubSystem2533/SubSystem2547/SubSystem2550 ==
  note: ***編集禁止***
  input : Inport
  element : Inport  Port=2
  Assignment : Assignment  IndexOptions=Index vector (port)  OutputSizes=[1 1]
  Inside_DSR : DataStoreRead  DataStoreName=DSM289
  Inside_DSW : DataStoreWrite  DataStoreName=DSM289
  wires:
  element/1 -> Assignment/3
  input/1 -> Assignment/2
  Inside_DSR/1 -> Assignment/1  "mdl4_SubSystem2493_SubSystem2494_SubSystem2500_SubSystem2504_SubSystem2533_SubSystem2547_SubSystem2550_Inside_DSR_1"
  Assignment/1 -> Inside_DSW/1  "mdl4_SubSystem2493_SubSystem2494_SubSystem2500_SubSystem2504_SubSystem2533_SubSystem2547_SubSystem2550_Assignment_1"

== system mdl4/SubSystem2493/SubSystem2494/SubSystem2500/SubSystem2504/SubSystem2533/SubSystem2547/SubSystem2551 ==
  note: ***編集禁止***
  input : Inport
  element : Inport  Port=2
  Assignment : Assignment  IndexOptions=Index vector (port)  OutputSizes=[1 1]
  Inside_DSR : DataStoreRead  DataStoreName=DSM291
  Inside_DSW : DataStoreWrite  DataStoreName=DSM291
  wires:
  Assignment/1 -> Inside_DSW/1  "mdl4_SubSystem2493_SubSystem2494_SubSystem2500_SubSystem2504_SubSystem2533_SubSystem2547_SubSystem2551_Assignment_1"
  Inside_DSR/1 -> Assignment/1  "mdl4_SubSystem2493_SubSystem2494_SubSystem2500_SubSystem2504_SubSystem2533_SubSystem2547_SubSystem2551_Inside_DSR_1"
  input/1 -> Assignment/2
  element/1 -> Assignment/3

== system mdl4/SubSystem2493/SubSystem2494/SubSystem2500/SubSystem2504/SubSystem2533/SubSystem2547/SubSystem2552 ==
  note: ***編集禁止***
  mult : Inport
  div : Inport  Port=2
  Product : Product  Inputs=*/  SaturateOnIntegerOverflow=on  RndMeth=Zero  InputSameDT=on  OutDataTypeStr=Inherit: Same as first input
  Out : Outport
  wires:
  Product/1 -> Out/1  "mdl4_SubSystem2493_SubSystem2494_SubSystem2500_SubSystem2504_SubSystem2533_SubSystem2547_SubSystem2552_Product_1"
  mult/1 -> Product/1
  div/1 -> Product/2

== system mdl4/SubSystem2493/SubSystem2494/SubSystem2500/SubSystem2504/SubSystem2533/SubSystem2547/SubSystem2553 ==
  note: ***編集禁止***
  N : Inport
  For_loop : Stateflow chart  TreatAsAtomicUnit=on
  action : Outport
  i : Outport  Port=2
  wires:
  For_loop/1(idx) -> i/1
  N/1 -> For_loop/1(N_Loop)
  For_loop/2(function_call) -> action/1

== system mdl4/SubSystem2493/SubSystem2494/SubSystem2500/SubSystem2504/SubSystem2533/SubSystem2547/SubSystem2554 ==
  note: Text645
  note: Text644
  note: Text643
  note: Text642
  note: Text641
  Block7642 : Inport
  Block7643 : TriggerPort  TriggerType=function-call
  Block7644 : DataStoreRead  DataStoreName=DSM288
  Block7645 : DataStoreRead  DataStoreName=DSM287
  Block7646 : DataStoreWrite  DataStoreName=DSM288
  Block7647 : DataStoreWrite  DataStoreName=DSM287
  Block7648 : Sum  Inputs=++|  OutDataTypeStr=double  RndMeth=Zero  SaturateOnIntegerOverflow=on  InputSameDT=on
  Block7649 : Sum  Inputs=++|  OutDataTypeStr=double  RndMeth=Zero  SaturateOnIntegerOverflow=on  InputSameDT=on
  SubSystem2555 : Subsystem  TreatAsAtomicUnit=on  mask(***ATC.DSRVEC***){bd_version=1.01.A, r0=DSM293, r1=-1, r2=, r3=, r4=, r5=, r6=, r7=, r8=, r9=, c0=, c1=, c2=, c3=, c4=, c5=, c6=, c7=, c8=, c9=}
      mask prompts: bd_version "Version"
      mask help: これはAutoCからのブロックです．編集禁止．
      settings: OpenFcn=warndlg('変更禁止!');
      mask Help: web(ui_blockhelpmng(gcb));
      mask Display: disp('ATC.DSRVEC')
  SubSystem2556 : Subsystem  TreatAsAtomicUnit=on  mask(***ATC.DSRVEC***){bd_version=1.01.A, r0=DSM295, r1=-1, r2=, r3=, r4=, r5=, r6=, r7=, r8=, r9=, c0=, c1=, c2=, c3=, c4=, c5=, c6=, c7=, c8=, c9=}
      mask prompts: bd_version "Version"
      mask help: これはAutoCからのブロックです．編集禁止．
      settings: OpenFcn=warndlg('変更禁止!');
      mask Help: web(ui_blockhelpmng(gcb));
      mask Display: disp('ATC.DSRVEC')
  wires:
  Block7648/1 -> Block7646/1  "mdl4_SubSystem2493_SubSystem2494_SubSystem2500_SubSystem2504_SubSystem2533_SubSystem2547_SubSystem2554_Block7648_1"
  Block7644/1 -> Block7648/1  "mdl4_SubSystem2493_SubSystem2494_SubSystem2500_SubSystem2504_SubSystem2533_SubSystem2547_SubSystem2554_Block7644_1"
  Block7649/1 -> Block7647/1  "mdl4_SubSystem2493_SubSystem2494_SubSystem2500_SubSystem2504_SubSystem2533_SubSystem2547_SubSystem2554_Block7649_1"
  Block7645/1 -> Block7649/1  "mdl4_SubSystem2493_SubSystem2494_SubSystem2500_SubSystem2504_SubSystem2533_SubSystem2547_SubSystem2554_Block7645_1"
  SubSystem2555/1(Output) -> Block7649/2  "mdl4_SubSystem2493_SubSystem2494_SubSystem2500_SubSystem2504_SubSystem2533_SubSystem2547_SubSystem2554_SubSystem2555_SigLabel295"
  Block7642/1 -> SubSystem2555/1(element), SubSystem2556/1(element)
  SubSystem2556/1(Output) -> Block7648/2  "mdl4_SubSystem2493_SubSystem2494_SubSystem2500_SubSystem2504_SubSystem2533_SubSystem2547_SubSystem2554_SubSystem2556_SigLabel294"

== system mdl4/SubSystem2493/SubSystem2494/SubSystem2500/SubSystem2504/SubSystem2533/SubSystem2557/SubSystem2558 ==
  note: ***編集禁止***
  input : Inport
  element : Inport  Port=2
  Assignment : Assignment  IndexOptions=Index vector (port)  OutputSizes=[1 1]
  Inside_DSR : DataStoreRead  DataStoreName=DSM290
  Inside_DSW : DataStoreWrite  DataStoreName=DSM290
  wires:
  element/1 -> Assignment/3
  input/1 -> Assignment/2
  Inside_DSR/1 -> Assignment/1  "mdl4_SubSystem2493_SubSystem2494_SubSystem2500_SubSystem2504_SubSystem2533_SubSystem2557_SubSystem2558_Inside_DSR_1"
  Assignment/1 -> Inside_DSW/1  "mdl4_SubSystem2493_SubSystem2494_SubSystem2500_SubSystem2504_SubSystem2533_SubSystem2557_SubSystem2558_Assignment_1"

== system mdl4/SubSystem2493/SubSystem2494/SubSystem2500/SubSystem2504/SubSystem2533/SubSystem2557/SubSystem2559 ==
  note: ***編集禁止***
  input : Inport
  element : Inport  Port=2
  Assignment : Assignment  IndexOptions=Index vector (port)  OutputSizes=[1 1]
  Inside_DSR : DataStoreRead  DataStoreName=DSM292
  Inside_DSW : DataStoreWrite  DataStoreName=DSM292
  wires:
  Assignment/1 -> Inside_DSW/1  "mdl4_SubSystem2493_SubSystem2494_SubSystem2500_SubSystem2504_SubSystem2533_SubSystem2557_SubSystem2559_Assignment_1"
  Inside_DSR/1 -> Assignment/1  "mdl4_SubSystem2493_SubSystem2494_SubSystem2500_SubSystem2504_SubSystem2533_SubSystem2557_SubSystem2559_Inside_DSR_1"
  input/1 -> Assignment/2
  element/1 -> Assignment/3

== system mdl4/SubSystem2493/SubSystem2494/SubSystem2500/SubSystem2504/SubSystem2533/SubSystem2557/SubSystem2560 ==
  note: ***編集禁止***
  input : Inport
  element : Inport  Port=2
  Assignment : Assignment  IndexOptions=Index vector (port)  OutputSizes=[1 1]
  Inside_DSR : DataStoreRead  DataStoreName=DSM289
  Inside_DSW : DataStoreWrite  DataStoreName=DSM289
  wires:
  Assignment/1 -> Inside_DSW/1  "mdl4_SubSystem2493_SubSystem2494_SubSystem2500_SubSystem2504_SubSystem2533_SubSystem2557_SubSystem2560_Assignment_1"
  Inside_DSR/1 -> Assignment/1  "mdl4_SubSystem2493_SubSystem2494_SubSystem2500_SubSystem2504_SubSystem2533_SubSystem2557_SubSystem2560_Inside_DSR_1"
  input/1 -> Assignment/2
  element/1 -> Assignment/3

== system mdl4/SubSystem2493/SubSystem2494/SubSystem2500/SubSystem2504/SubSystem2533/SubSystem2557/SubSystem2561 ==
  note: ***編集禁止***
  input : Inport
  element : Inport  Port=2
  Assignment : Assignment  IndexOptions=Index vector (port)  OutputSizes=[1 1]
  Inside_DSR : DataStoreRead  DataStoreName=DSM291
  Inside_DSW : DataStoreWrite  DataStoreName=DSM291
  wires:
  element/1 -> Assignment/3
  input/1 -> Assignment/2
  Inside_DSR/1 -> Assignment/1  "mdl4_SubSystem2493_SubSystem2494_SubSystem2500_SubSystem2504_SubSystem2533_SubSystem2557_SubSystem2561_Inside_DSR_1"
  Assignment/1 -> Inside_DSW/1  "mdl4_SubSystem2493_SubSystem2494_SubSystem2500_SubSystem2504_SubSystem2533_SubSystem2557_SubSystem2561_Assignment_1"

== system mdl4/SubSystem2493/SubSystem2494/SubSystem2500/SubSystem2504/SubSystem2533/SubSystem2557/SubSystem2562 ==
  note: ***編集禁止***
  mult : Inport
  div : Inport  Port=2
  Product : Product  Inputs=*/  SaturateOnIntegerOverflow=on  RndMeth=Zero  InputSameDT=on  OutDataTypeStr=Inherit: Same as first input
  Out : Outport
  wires:
  div/1 -> Product/2
  mult/1 -> Product/1
  Product/1 -> Out/1  "mdl4_SubSystem2493_SubSystem2494_SubSystem2500_SubSystem2504_SubSystem2533_SubSystem2557_SubSystem2562_Product_1"

== system mdl4/SubSystem2493/SubSystem2494/SubSystem2500/SubSystem2504/SubSystem2533/SubSystem2557/SubSystem2563 ==
  note: ***編集禁止***
  N : Inport
  For_loop : Stateflow chart  TreatAsAtomicUnit=on
  action : Outport
  i : Outport  Port=2
  wires:
  For_loop/1(idx) -> i/1
  N/1 -> For_loop/1(N_Loop)
  For_loop/2(function_call) -> action/1

== system mdl4/SubSystem2493/SubSystem2494/SubSystem2500/SubSystem2504/SubSystem2533/SubSystem2557/SubSystem2564 ==
  note: Text655
  note: Text654
  note: Text653
  note: Text652
  note: Text651
  Block7668 : Inport
  Block7669 : TriggerPort  TriggerType=function-call
  Block7670 : DataStoreRead  DataStoreName=DSM288
  Block7671 : DataStoreRead  DataStoreName=DSM287
  Block7672 : DataStoreWrite  DataStoreName=DSM288
  Block7673 : DataStoreWrite  DataStoreName=DSM287
  Block7674 : Sum  Inputs=++|  OutDataTypeStr=double  RndMeth=Zero  SaturateOnIntegerOverflow=on  InputSameDT=on
  Block7675 : Sum  Inputs=++|  OutDataTypeStr=double  RndMeth=Zero  SaturateOnIntegerOverflow=on  InputSameDT=on
  SubSystem2565 : Subsystem  TreatAsAtomicUnit=on  mask(***ATC.DSRVEC***){bd_version=1.01.A, r0=DSM279, r1=-1, r2=, r3=, r4=, r5=, r6=, r7=, r8=, r9=, c0=, c1=, c2=, c3=, c4=, c5=, c6=, c7=, c8=, c9=}
      mask prompts: bd_version "Version"
      mask help: これはAutoCからのブロックです．編集禁止．
      settings: OpenFcn=warndlg('変更禁止!');
      mask Help: web(ui_blockhelpmng(gcb));
      mask Display: disp('ATC.DSRVEC')
  SubSystem2566 : Subsystem  TreatAsAtomicUnit=on  mask(***ATC.DSRVEC***){bd_version=1.01.A, r0=DSM280, r1=-1, r2=, r3=, r4=, r5=, r6=, r7=, r8=, r9=, c0=, c1=, c2=, c3=, c4=, c5=, c6=, c7=, c8=, c9=}
      mask prompts: bd_version "Version"
      mask help: これはAutoCからのブロックです．編集禁止．
      settings: OpenFcn=warndlg('変更禁止!');
      mask Help: web(ui_blockhelpmng(gcb));
      mask Display: disp('ATC.DSRVEC')
  wires:
  SubSystem2566/1(Output) -> Block7674/2  "mdl4_SubSystem2493_SubSystem2494_SubSystem2500_SubSystem2504_SubSystem2533_SubSystem2557_SubSystem2564_SubSystem2566_SigLabel297"
  Block7668/1 -> SubSystem2565/1(element), SubSystem2566/1(element)
  SubSystem2565/1(Output) -> Block7675/2  "mdl4_SubSystem2493_SubSystem2494_SubSystem2500_SubSystem2504_SubSystem2533_SubSystem2557_SubSystem2564_SubSystem2565_SigLabel296"
  Block7671/1 -> Block7675/1  "mdl4_SubSystem2493_SubSystem2494_SubSystem2500_SubSystem2504_SubSystem2533_SubSystem2557_SubSystem2564_Block7671_1"
  Block7675/1 -> Block7673/1  "mdl4_SubSystem2493_SubSystem2494_SubSystem2500_SubSystem2504_SubSystem2533_SubSystem2557_SubSystem2564_Block7675_1"
  Block7670/1 -> Block7674/1  "mdl4_SubSystem2493_SubSystem2494_SubSystem2500_SubSystem2504_SubSystem2533_SubSystem2557_SubSystem2564_Block7670_1"
  Block7674/1 -> Block7672/1  "mdl4_SubSystem2493_SubSystem2494_SubSystem2500_SubSystem2504_SubSystem2533_SubSystem2557_SubSystem2564_Block7674_1"

== system mdl4/SubSystem2493/SubSystem2494/SubSystem2500/SubSystem2504/SubSystem2533/SubSystem2567/SubSystem2568 ==
  note: ***編集禁止***
  input : Inport
  element : Inport  Port=2
  Assignment : Assignment  IndexOptions=Index vector (port)  OutputSizes=[1 1]
  Inside_DSR : DataStoreRead  DataStoreName=DSM290
  Inside_DSW : DataStoreWrite  DataStoreName=DSM290
  wires:
  Assignment/1 -> Inside_DSW/1  "mdl4_SubSystem2493_SubSystem2494_SubSystem2500_SubSystem2504_SubSystem2533_SubSystem2567_SubSystem2568_Assignment_1"
  Inside_DSR/1 -> Assignment/1  "mdl4_SubSystem2493_SubSystem2494_SubSystem2500_SubSystem2504_SubSystem2533_SubSystem2567_SubSystem2568_Inside_DSR_1"
  input/1 -> Assignment/2
  element/1 -> Assignment/3

== system mdl4/SubSystem2493/SubSystem2494/SubSystem2500/SubSystem2504/SubSystem2533/SubSystem2567/SubSystem2569 ==
  note: ***編集禁止***
  input : Inport
  element : Inport  Port=2
  Assignment : Assignment  IndexOptions=Index vector (port)  OutputSizes=[1 1]
  Inside_DSR : DataStoreRead  DataStoreName=DSM292
  Inside_DSW : DataStoreWrite  DataStoreName=DSM292
  wires:
  element/1 -> Assignment/3
  input/1 -> Assignment/2
  Inside_DSR/1 -> Assignment/1  "mdl4_SubSystem2493_SubSystem2494_SubSystem2500_SubSystem2504_SubSystem2533_SubSystem2567_SubSystem2569_Inside_DSR_1"
  Assignment/1 -> Inside_DSW/1  "mdl4_SubSystem2493_SubSystem2494_SubSystem2500_SubSystem2504_SubSystem2533_SubSystem2567_SubSystem2569_Assignment_1"

== system mdl4/SubSystem2493/SubSystem2494/SubSystem2500/SubSystem2504/SubSystem2533/SubSystem2567/SubSystem2570 ==
  note: ***編集禁止***
  input : Inport
  element : Inport  Port=2
  Assignment : Assignment  IndexOptions=Index vector (port)  OutputSizes=[1 1]
  Inside_DSR : DataStoreRead  DataStoreName=DSM289
  Inside_DSW : DataStoreWrite  DataStoreName=DSM289
  wires:
  element/1 -> Assignment/3
  input/1 -> Assignment/2
  Inside_DSR/1 -> Assignment/1  "mdl4_SubSystem2493_SubSystem2494_SubSystem2500_SubSystem2504_SubSystem2533_SubSystem2567_SubSystem2570_Inside_DSR_1"
  Assignment/1 -> Inside_DSW/1  "mdl4_SubSystem2493_SubSystem2494_SubSystem2500_SubSystem2504_SubSystem2533_SubSystem2567_SubSystem2570_Assignment_1"

== system mdl4/SubSystem2493/SubSystem2494/SubSystem2500/SubSystem2504/SubSystem2533/SubSystem2567/SubSystem2571 ==
  note: ***編集禁止***
  input : Inport
  element : Inport  Port=2
  Assignment : Assignment  IndexOptions=Index vector (port)  OutputSizes=[1 1]
  Inside_DSR : DataStoreRead  DataStoreName=DSM291
  Inside_DSW : DataStoreWrite  DataStoreName=DSM291
  wires:
  Assignment/1 -> Inside_DSW/1  "mdl4_SubSystem2493_SubSystem2494_SubSystem2500_SubSystem2504_SubSystem2533_SubSystem2567_SubSystem2571_Assignment_1"
  Inside_DSR/1 -> Assignment/1  "mdl4_SubSystem2493_SubSystem2494_SubSystem2500_SubSystem2504_SubSystem2533_SubSystem2567_SubSystem2571_Inside_DSR_1"
  input/1 -> Assignment/2
  element/1 -> Assignment/3

== system mdl4/SubSystem2493/SubSystem2494/SubSystem2500/SubSystem2504/SubSystem2533/SubSystem2567/SubSystem2572 ==
  note: ***編集禁止***
  mult : Inport
  div : Inport  Port=2
  Product : Product  Inputs=*/  SaturateOnIntegerOverflow=on  RndMeth=Zero  InputSameDT=on  OutDataTypeStr=Inherit: Same as first input
  Out : Outport
  wires:
  Product/1 -> Out/1  "mdl4_SubSystem2493_SubSystem2494_SubSystem2500_SubSystem2504_SubSystem2533_SubSystem2567_SubSystem2572_Product_1"
  mult/1 -> Product/1
  div/1 -> Product/2

== system mdl4/SubSystem2493/SubSystem2494/SubSystem2500/SubSystem2504/SubSystem2533/SubSystem2567/SubSystem2573 ==
  note: ***編集禁止***
  N : Inport
  For_loop : Stateflow chart  TreatAsAtomicUnit=on
  action : Outport
  i : Outport  Port=2
  wires:
  For_loop/1(idx) -> i/1
  N/1 -> For_loop/1(N_Loop)
  For_loop/2(function_call) -> action/1
